simulink model "controller"  (R2023b)
settings: Solver=VariableStepAuto  StartTime=0.0  StopTime=10.0  RelTol=1e-3
undefined symbols (not defined in the file or in its folder): K
settings Model: Creator=paoli  LastModifiedBy=kiraa

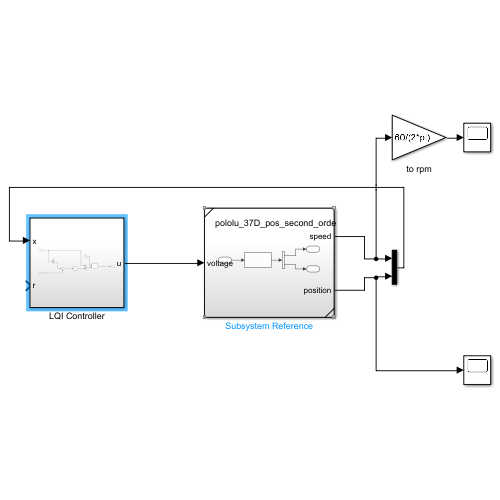
[thumbnail: Simulink's stored preview of the top-level diagram]
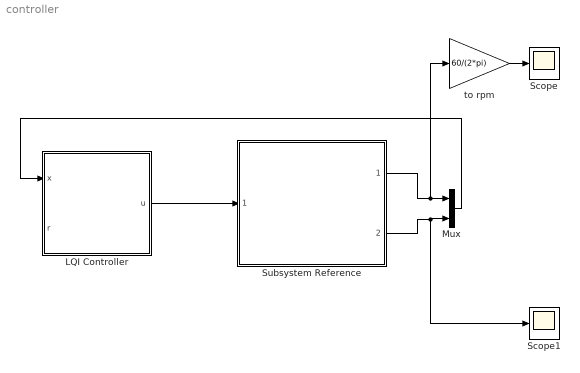
== system controller ==
  LQI Controller : Subsystem
  Mux : Mux  Inputs=2
  Scope : Scope
  Scope1 : Scope
  Subsystem Reference : Subsystem  ReferencedSubsystem=pololu_37D_pos_second_order
  to rpm : Gain  Gain=60/(2*pi)
  wires:
  Mux/1 -> LQI Controller/1(x)
  LQI Controller/1(u) -> Subsystem Reference/1
  Subsystem Reference/1 -> to rpm/1, Mux/1
  Subsystem Reference/2 -> Mux/2, Scope1/1
  to rpm/1 -> Scope/1

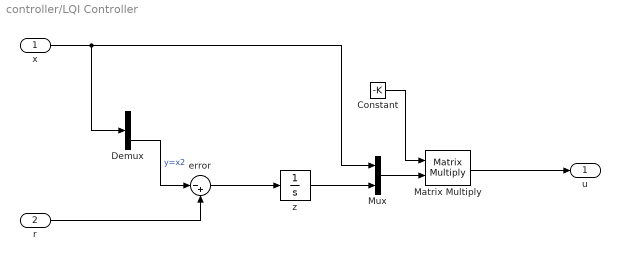
== system controller/LQI Controller ==
  x : Inport
  r : Inport  Port=2
  Constant : Constant  Value=-K  VectorParams1D=off
  Demux : Demux  Outputs=2
  Matrix Multiply : Product  Multiplication=Matrix(*)
  Mux : Mux  Inputs=2
  error : Sum  Inputs=|-+
  z : Integrator  InitialCondition=0.1
  u : Outport
  wires:
  Constant/1 -> Matrix Multiply/1
  Matrix Multiply/1 -> u/1
  x/1 -> Mux/1, Demux/1
  Mux/1 -> Matrix Multiply/2
  error/1 -> z/1
  r/1 -> error/2
  z/1 -> Mux/2
  Demux/2 -> error/1  "y=x2"
